simulink model "Table_airbus_v1"  (R2021b)
settings: Solver=VariableStepAuto  StartTime=0.0  StopTime=20  MaxStep=0.01  RelTol=0.01
undefined symbols (not defined in the file): X, Y, Z
libraries: sm_lib x907, fl_lib x69, nesl_utility x53, sdl_lib x10, ee_lib x7, slpidlib x6, simulink x5, simulink_extras x4
(part 2 of 18)

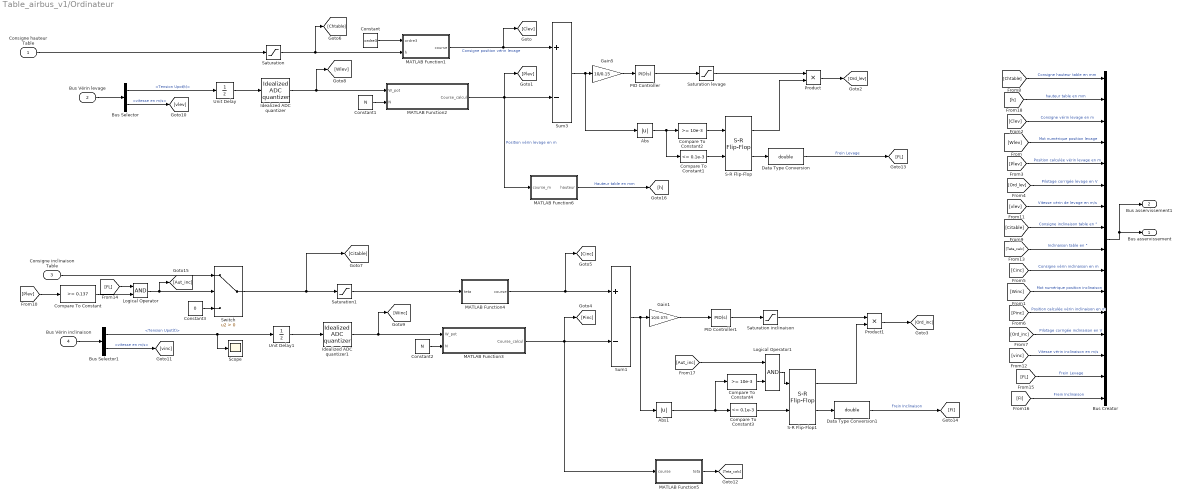
== system Table_airbus_v1/Ordinateur ==
  Consigne hauteur Table : Inport
  Bus Vérin levage : Inport  Port=2
  Consigne inclinaison Table : Inport  Port=3
  Bus Vérin inclinaison : Inport  Port=4
  Abs : Abs
  Abs1 : Abs
  Bus Creator : BusCreator  Inputs=16
  Bus Selector : BusSelector  OutputSignals=Tension Upot(t),Bus vis écrou.vitesse en m/s
  Bus Selector1 : BusSelector  OutputSignals=Tension Upot(t),Bus vis écrou.vitesse en m/s
  Compare To Constant : simulink/Logic and Bit Operations/Compare To Constant  relop=>=  const=0.137  OutDataTypeStr=boolean
  Compare To Constant1 : simulink/Logic and Bit Operations/Compare To Constant  relop=<=  const=0.1e-3  OutDataTypeStr=boolean
  Compare To Constant2 : simulink/Logic and Bit Operations/Compare To Constant  relop=>=  const=10e-3  OutDataTypeStr=boolean
  Compare To Constant3 : simulink/Logic and Bit Operations/Compare To Constant  relop=<=  const=0.1e-3  OutDataTypeStr=boolean
  Compare To Constant4 : simulink/Logic and Bit Operations/Compare To Constant  relop=>=  const=10e-3  OutDataTypeStr=boolean
  Constant : Constant  Value=ordre3
  Constant1 : Constant  Value=N
  Constant2 : Constant  Value=N
  Constant3 : Constant  Value=0
  Data Type Conversion : DataTypeConversion  OutDataTypeStr=double
  Data Type Conversion1 : DataTypeConversion  OutDataTypeStr=double
  Gain1 : Gain  Gain=10/0.075
  Gain5 : Gain  Gain=10/0.15
  Idealized ADC quantizer : simulink_extras/Additional Discrete/Idealized ADC quantizer  NumberOfConverterBits=N  Vmin=-10  Vmax=10  OutputDataType=int16  OutputNegativeValues=on
  Idealized ADC quantizer1 : simulink_extras/Additional Discrete/Idealized ADC quantizer  NumberOfConverterBits=N  Vmin=-10  Vmax=10  OutputDataType=int16  OutputNegativeValues=on
  Logical Operator : Logic  AllPortsSameDT=off  OutDataTypeStr=boolean
  Logical Operator1 : Logic  AllPortsSameDT=off  OutDataTypeStr=boolean
  MATLAB Function1 : MATLAB Function  TreatAsAtomicUnit=on
  MATLAB Function2 : MATLAB Function  TreatAsAtomicUnit=on
  MATLAB Function3 : MATLAB Function  TreatAsAtomicUnit=on
  MATLAB Function4 : MATLAB Function  TreatAsAtomicUnit=on
  MATLAB Function5 : MATLAB Function  TreatAsAtomicUnit=on
  MATLAB Function6 : MATLAB Function  TreatAsAtomicUnit=on
  PID Controller : slpidlib/PID Controller  Controller=PID  Form=Parallel  TimeDomain=Continuous-time  UseExternalTs=off  SampleTime=-1  IntegratorMethod=Forward Euler  FilterMethod=Forward Euler  ControllerParametersSource=internal  P=kp_lev  I=ki_lev  D=kd_lev  UseFilter=on  N=10  TunerSelectOption=Transfer Function Based (PID Tuner App)  InitialConditionSource=internal  InitialConditionForIntegrator=0  InitialConditionForFilter=0  DifferentiatorICPrevScaledInput=0  ExternalReset=none  TrackingMode=off  Kt=1  LimitOutput=off  SatLimitsSource=internal  UpperSaturationLimit=inf  LowerSaturationLimit=-inf  LinearizeAsGain=on  AntiWindupMode=none  Kb=1  POutMin=[]  POutMax=[]  IOutMin=[]  IOutMax=[]  DOutMin=[]  DOutMax=[]  NOutMin=[]  NOutMax=[]  SumOutMin=[]  SumOutMax=[]  SaturationOutMin=[]  SaturationOutMax=[]  PParamMin=[]  PParamMax=[]  IParamMin=[]  IParamMax=[]  DParamMin=[]  DParamMax=[]  NParamMin=[]  NParamMax=[]  KbParamMin=[]  KbParamMax=[]  KtParamMin=[]  KtParamMax=[]  KbOutMin=[]  KbOutMax=[]  KtOutMin=[]  KtOutMax=[]  IntegratorOutMin=[]  IntegratorOutMax=[]  FilterOutMin=[]  FilterOutMax=[]  SumI1OutMin=[]  SumI1OutMax=[]  SumI2OutMin=[]  SumI2OutMax=[]  SumI3OutMin=[]  SumI3OutMax=[]  SumI4OutMin=[]  SumI4OutMax=[]  SumDOutMin=[]  SumDOutMax=[]  DifferentiatorOutMin=[]  DifferentiatorOutMax=[]  FilterDiffOutCoefMin=[]  FilterDiffOutCoefMax=[]  ReciprocalOutMin=[]  ReciprocalOutMax=[]  SumDenOutMin=[]  SumDenOutMax=[]  SumNumOutMin=[]  SumNumOutMax=[]  DivideOutMin=[]  DivideOutMax=[]  UdiffTsProdOutMin=[]  UdiffTsProdOutMax=[]  NTsProdOutMin=[]  NTsProdOutMax=[]  UintegralTsProdOutMin=[]  UintegralTsProdOutMax=[]  UngainTsProdOutMin=[]  UngainTsProdOutMax=[]  IntegratorContinuousStateAttributes=''  IntegratorStateMustResolveToSignalObject=off  IntegratorRTWStateStorageClass=Auto  FilterContinuousStateAttributes=''  FilterStateMustResolveToSignalObject=off  FilterRTWStateStorageClass=Auto  ParallelPVariant=InternalParameters  IdealPVariant=Disabled  IVariant=InternalParameters  DVariant=InternalParameters  IntegratorVariant=Continuous  SatVariant=Disabled  AWVariant=Passthrough  PCopyVariant=Disabled  TRVariant=Disabled  FdbkBlocksVariant=Forward  IdealPFdbkVariant=Disabled  SatFdbkVariant=Disabled  DerivativeFilterVariant=ContFilter  NVariant=InternalParameters  NCopyVariant=Disabled  FilterICVariant=InternalICsFilter  IntegratorICVariant=InternalICs  ExternalResetVariant=Disabled  TRSumVariant=Passthrough  SumFdbkVariant=Disabled  SumVariant=Sum_PID  TsampFilterVariant=InternalTs  TsampNgainVariant=Passthrough  TsampIntegralVariant=Passthrough  ExternalSaturationOutDataTypeStr=Inherit: Same as second input
  PID Controller1 : slpidlib/PID Controller  Controller=PID  Form=Parallel  TimeDomain=Continuous-time  UseExternalTs=off  SampleTime=1  IntegratorMethod=Forward Euler  FilterMethod=Forward Euler  ControllerParametersSource=internal  P=kp_inc  I=ki_inc  D=kd_inc  UseFilter=on  N=10  TunerSelectOption=Transfer Function Based (PID Tuner App)  InitialConditionSource=internal  InitialConditionForIntegrator=0  InitialConditionForFilter=0  DifferentiatorICPrevScaledInput=0  ExternalReset=none  TrackingMode=off  Kt=1  LimitOutput=off  SatLimitsSource=internal  UpperSaturationLimit=inf  LowerSaturationLimit=-inf  LinearizeAsGain=on  AntiWindupMode=none  Kb=1  POutMin=[]  POutMax=[]  IOutMin=[]  IOutMax=[]  DOutMin=[]  DOutMax=[]  NOutMin=[]  NOutMax=[]  SumOutMin=[]  SumOutMax=[]  SaturationOutMin=[]  SaturationOutMax=[]  PParamMin=[]  PParamMax=[]  IParamMin=[]  IParamMax=[]  DParamMin=[]  DParamMax=[]  NParamMin=[]  NParamMax=[]  KbParamMin=[]  KbParamMax=[]  KtParamMin=[]  KtParamMax=[]  KbOutMin=[]  KbOutMax=[]  KtOutMin=[]  KtOutMax=[]  IntegratorOutMin=[]  IntegratorOutMax=[]  FilterOutMin=[]  FilterOutMax=[]  SumI1OutMin=[]  SumI1OutMax=[]  SumI2OutMin=[]  SumI2OutMax=[]  SumI3OutMin=[]  SumI3OutMax=[]  SumI4OutMin=[]  SumI4OutMax=[]  SumDOutMin=[]  SumDOutMax=[]  DifferentiatorOutMin=[]  DifferentiatorOutMax=[]  FilterDiffOutCoefMin=[]  FilterDiffOutCoefMax=[]  ReciprocalOutMin=[]  ReciprocalOutMax=[]  SumDenOutMin=[]  SumDenOutMax=[]  SumNumOutMin=[]  SumNumOutMax=[]  DivideOutMin=[]  DivideOutMax=[]  UdiffTsProdOutMin=[]  UdiffTsProdOutMax=[]  NTsProdOutMin=[]  NTsProdOutMax=[]  UintegralTsProdOutMin=[]  UintegralTsProdOutMax=[]  UngainTsProdOutMin=[]  UngainTsProdOutMax=[]  IntegratorContinuousStateAttributes=''  IntegratorStateMustResolveToSignalObject=off  IntegratorRTWStateStorageClass=Auto  FilterContinuousStateAttributes=''  FilterStateMustResolveToSignalObject=off  FilterRTWStateStorageClass=Auto  ParallelPVariant=InternalParameters  IdealPVariant=Disabled  IVariant=InternalParameters  DVariant=InternalParameters  IntegratorVariant=Continuous  SatVariant=Disabled  AWVariant=Passthrough  PCopyVariant=Disabled  TRVariant=Disabled  FdbkBlocksVariant=Forward  IdealPFdbkVariant=Disabled  SatFdbkVariant=Disabled  DerivativeFilterVariant=ContFilter  NVariant=InternalParameters  NCopyVariant=Disabled  FilterICVariant=InternalICsFilter  IntegratorICVariant=InternalICs  ExternalResetVariant=Disabled  TRSumVariant=Passthrough  SumFdbkVariant=Disabled  SumVariant=Sum_PID  TsampFilterVariant=InternalTs  TsampNgainVariant=Passthrough  TsampIntegralVariant=Passthrough  ExternalSaturationOutDataTypeStr=Inherit: Same as second input
  Product : Product
  Product1 : Product
  S-R Flip-Flop : simulink_extras/Flip Flops/S-R Flip-Flop  initial_condition=0
  S-R Flip-Flop1 : simulink_extras/Flip Flops/S-R Flip-Flop  initial_condition=0
  Saturation : Saturate  UpperLimit=pos_lev_max  LowerLimit=pos_lev_min
  Saturation inclinaison : Saturate  UpperLimit=10  LowerLimit=-10
  Saturation levage : Saturate  UpperLimit=10  LowerLimit=-10
  Saturation1 : Saturate  UpperLimit=20  LowerLimit=-20
  Scope : Scope
  Sum1 : Sum  Inputs=+-
  Sum3 : Sum  Inputs=+-
  Switch : Switch  Criteria=u2 > Threshold
  Unit Delay : UnitDelay  SampleTime=-1  HasFrameUpgradeWarning=on
  Unit Delay1 : UnitDelay  SampleTime=-1  HasFrameUpgradeWarning=on
  Bus asservissement : Outport  VectorParamsAs1DForOutWhenUnconnected=off
  Bus asservissement1 : Outport  Port=2  VectorParamsAs1DForOutWhenUnconnected=off
  wires:
  Saturation levage/1 -> Product/1
  Sum3/1 -> Abs/1, Gain5/1
  Consigne hauteur Table/1 -> Saturation/1
  MATLAB Function2/1(Course_calcul) -> MATLAB Function6/1(course_m), Sum3/2, [Plev]  "Position vérin levage en m"
  PID Controller/1 -> Saturation levage/1
  MATLAB Function3/1(Course_calcul) -> MATLAB Function5/1(course), [Pinc], Sum1/2
  MATLAB Function4/1(course) -> Sum1/1, [Cinc]
  Switch/1 -> [Citable], Saturation1/1
  Sum1/1 -> Abs1/1, Gain1/1
  MATLAB Function1/1(course) -> Sum3/1, [Clev]  "Consigne position vérin levage"
  Constant/1 -> MATLAB Function1/1(ordre3)
  Saturation/1 -> [Chtable], MATLAB Function1/2(h)
  [Clev] -> Bus Creator/3  "Consigne vérin levage en m"
  [Plev] -> Bus Creator/5  "Position calculée vérin levage en m"
  Bus Creator/1 -> Bus asservissement1/1, Bus asservissement/1
  [Ord_lev] -> Bus Creator/6  "Pilotage corrigée levage en V"
  [Ord_inc] -> Bus Creator/13  "Pilotage corrigée inclinaison en V"
  [Pinc] -> Bus Creator/12  "Position calculée vérin inclinaison en m"
  [Cinc] -> Bus Creator/10  "Consigne vérin inclinaison en m"
  [Chtable] -> Bus Creator/1  "Consigne hauteur table en mm"
  [Citable] -> Bus Creator/8  "Consigne inclinaison table en °"
  Bus Vérin inclinaison/1 -> Bus Selector1/1
  Constant1/1 -> MATLAB Function2/2(N)
  Gain5/1 -> PID Controller/1
  Constant2/1 -> MATLAB Function3/2(N)
  PID Controller1/1 -> Saturation inclinaison/1
  Gain1/1 -> PID Controller1/1
  Bus Selector1/1 -> Unit Delay1/1, Scope/1  "<Tension Upot(t)>"
  Bus Selector/1 -> Unit Delay/1  "<Tension Upot(t)>"
  Idealized ADC quantizer/1 -> [Wlev], MATLAB Function2/1(W_pot)
  [Wlev] -> Bus Creator/4  "Mot numérique position levage"
  Idealized ADC quantizer1/1 -> [Winc], MATLAB Function3/1(W_pot)
  Saturation1/1 -> MATLAB Function4/1(teta)
  [Winc] -> Bus Creator/11  "Mot numérique position inclinaison"
  [Plev] -> Compare To Constant/1
  Logical Operator/1 -> [Aut_inc], Switch/2
  Constant3/1 -> Switch/3
  Consigne inclinaison Table/1 -> Switch/1
  Unit Delay1/1 -> Idealized ADC quantizer1/1
  Bus Selector/2 -> [vlev]  "<vitesse en m/s>"
  [vlev] -> Bus Creator/7  "Vitesse vérin de levage en m/s"
  Unit Delay/1 -> Idealized ADC quantizer/1
  Bus Selector1/2 -> [vinc]  "<vitesse en m/s>"
  [vinc] -> Bus Creator/14  "Vitesse vérin inclinaison en m/s"
  MATLAB Function5/1(teta) -> [Teta_calc]
  [Teta_calc] -> Bus Creator/9  "Inclinaison table en °"
  Saturation inclinaison/1 -> Product1/1
  Data Type Conversion/1 -> [FL]  "Frein Levage"
  Compare To Constant2/1 -> S-R Flip-Flop/1
  Abs/1 -> Compare To Constant2/1, Compare To Constant1/1
  Bus Vérin levage/1 -> Bus Selector/1
  S-R Flip-Flop/2 -> Data Type Conversion/1
  Compare To Constant1/1 -> S-R Flip-Flop/2
  Product/1 -> [Ord_lev]
  S-R Flip-Flop/1 -> Product/2
  Compare To Constant/1 -> Logical Operator/2
  [FL] -> Logical Operator/1
  S-R Flip-Flop1/1 -> Product1/2
  S-R Flip-Flop1/2 -> Data Type Conversion1/1
  Data Type Conversion1/1 -> [FI]  "Frein Inclinaison"
  Product1/1 -> [Ord_inc]
  [FL] -> Bus Creator/15  "Frein Levage"
  [FI] -> Bus Creator/16  "Frein Inclinaison"
  [Aut_inc] -> Logical Operator1/1
  Abs1/1 -> Compare To Constant4/1, Compare To Constant3/1
  Compare To Constant3/1 -> S-R Flip-Flop1/2
  Logical Operator1/1 -> S-R Flip-Flop1/1
  Compare To Constant4/1 -> Logical Operator1/2
  MATLAB Function6/1(hauteur) -> [h]  "Hauteur table en mm"
  [h] -> Bus Creator/2  "hauteur table en mm"

== system Table_airbus_v1/Vérin électrique Inclinaison ==
  Pilotage Frein : Inport
  Bus Creator : BusCreator  Inputs=5
  Capteur : Subsystem
  Capteur mecanique Z1 : Subsystem
  Capteur mecanique Z2 : Subsystem
  Capteur mecanique Z3 : Subsystem
  Capteur mecanique Z4 : Subsystem
  Frein inclinaison : Subsystem
  Leadscrew : sdl_lib/Gears/Rotational- Translational/Leadscrew  Lead=pas_vis mm  helix_type=1  friction_model=2  friction_parameterization=1  lambda=Landa deg  alpha=Alpha deg  fr_coeff=fv  eff_sn=0.75  eff_ns=0.45  temperature_TLU=[280, 300, 320] K  efficiency_sn_TLU=[.75, .65, .6]  efficiency_ns_TLU=[.5, .45, .4]  pwr_thr=0.001 W  mu_visc=0 N*m/(rad/s)  thermal_mass=50 J/K  temperature_specify=off  temperature_priority=High  temperature=300 K  temperature_nominal_specify=off  temperature_nominal_unit=K  temperature_nominal_value=1
      settings: SourceProductBaseCode=LD  InternalSimscapePortConfiguration="{\"Bottom\":[],\"Left\":[{\"id\":\"S\",\"label\":\"S\",\"type\":\"foundation.mechanical.rotational.rotational\"}],\"Right\":[{\"id\":\"N\",\"label\":\"N\",\"type\":\"foundation.mechanical.translational.translational\"}],\"Top\":[]}"
  Mechanical Rotational Reference : fl_lib/Mechanical/Rotational Elements/Mechanical Rotational Reference
  Moteur : ee_lib/Electromechanical/Brushed Motors/DC Motor  field_option=ee.enum.field_option.pm  Rf=100 Ohm  Lf=1 H  Laf=0.15 H  If0=0 A  parameterization=1  Ra=R Ohm  La=L uH  emf_or_torque=2  Kv=0.0637 V/rpm  Ki=kt N*m/A  T_stall=3e-3*4000/(2*pi*6.25) N*m  w_max=3250 rpm  w_rated=2375 rpm  P_rated=19 W  V_rated=24 V  lam_param=2  i_noload=I0 A  V_i_noload=U0 V  J=Jm kg*m^2  lam=1e-08 N*m/(rad/s)  speed0=0 rpm  enable_fault_armature=simscape.enum.onoff.off  rev_faulted=1 / 3  G_faulted_armature=1e-5 S  fault_trigger_armature=ee.enum.faults.faultTrigger.temporal  t_fault_armature=1 s  max_permissible_current_armature=inf A  t_fail_on_current_armature=1 s  enable_fault_field=simscape.enum.onoff.off  G_faulted_field=1e-5 S  fault_trigger_field=ee.enum.faults.faultTrigger.temporal  t_fault_field=1 s  max_permissible_current_field=inf A  t_fail_on_current_field=1 s  fault_action=simscape.enum.assert.action.none  alpha=3.93e-3 1/K  Tmeas=25 degC  thermal_mass=100 J/K  initial_temperature=25 degC
  Scope : Scope
  réducteur train simple : sdl_lib/Gears/Simple Gear  ratio=ratio_red  rotation_direction=3-2*(1)  friction_model=sdl.enum.gear_efficiencies_load.constant  T_noload=0.1 N*m  T_nom=5 N*m  efficiency_nom=0.8  efficiency=rend_red/100  temperature_TLU=[280, 300, 320] K  load_TLU=[1, 5, 10] N*m  efficiency_TLU=[.95, .9, .85]  efficiency_TLU2=[.85, .8, .75; .95, .9, .85; .85, .8, .7]  w_thr=0.01 rad/s  pwr_thr=0.001 W  backlash_model=sdl.enum.backlashModel.Off  backlash_distance=1e-3 mm  x0=0 mm  r_base=0.1 m  hardstop_model=simscape.enum.hardstop.smooth  transition=1e-4 mm  backlash_stiffness=1e7 N/m  backlash_damping=1e6 N*s/m  e=0  v_tol=0.001 m/s  mu_visc=[0, 0] N*m/(rad/s)  enable_faults=simscape.enum.onoff.off  efficiency_fault=0.05  external_fault=simscape.enum.onoff.off  temporal_fault=simscape.enum.onoff.off  fault_time=5 s  fault_angles=pi / 12 rad  report_fault=(1)-1  thermal_mass=50 J/K  temperature_specify=off  temperature_priority=High  temperature=300 K  temperature_nominal_specify=off  temperature_nominal_unit=K  temperature_nominal_value=1  x_backlash_specify=off  x_backlash_priority=None  x_backlash=0 mm  x_backlash_nominal_specify=off  x_backlash_nominal_unit=mm  x_backlash_nominal_value=1  f_hardstop_specify=off  f_hardstop_priority=None  f_hardstop=0 N  f_hardstop_nominal_specify=off  f_hardstop_nominal_unit=N  f_hardstop_nominal_value=1  v_backlash_specify=off  v_backlash_priority=None  v_backlash=0 m/s  v_backlash_nominal_specify=off  v_backlash_nominal_unit=m/s  v_backlash_nominal_value=1
  réducteur train épicycloïdal : sdl_lib/Gears/Simple Gear  ratio=ratio_epi  rotation_direction=3-2*(1)  friction_model=sdl.enum.gear_efficiencies_load.constant  T_noload=0.1 N*m  T_nom=5 N*m  efficiency_nom=0.8  efficiency=rend_epi/100  temperature_TLU=[280, 300, 320] K  load_TLU=[1, 5, 10] N*m  efficiency_TLU=[.95, .9, .85]  efficiency_TLU2=[.85, .8, .75; .95, .9, .85; .85, .8, .7]  w_thr=0.01 rad/s  pwr_thr=0.001 W  backlash_model=sdl.enum.backlashModel.Off  backlash_distance=1e-3 mm  x0=0 mm  r_base=0.1 m  hardstop_model=simscape.enum.hardstop.smooth  transition=1e-4 mm  backlash_stiffness=1e7 N/m  backlash_damping=1e6 N*s/m  e=0  v_tol=0.001 m/s  mu_visc=[0, 0] N*m/(rad/s)  enable_faults=simscape.enum.onoff.off  efficiency_fault=0.05  external_fault=simscape.enum.onoff.off  temporal_fault=simscape.enum.onoff.off  fault_time=5 s  fault_angles=pi / 12 rad  report_fault=(1)-1  thermal_mass=50 J/K  temperature_specify=off  temperature_priority=High  temperature=300 K  temperature_nominal_specify=off  temperature_nominal_unit=K  temperature_nominal_value=1  x_backlash_specify=off  x_backlash_priority=None  x_backlash=0 mm  x_backlash_nominal_specify=off  x_backlash_nominal_unit=mm  x_backlash_nominal_value=1  f_hardstop_specify=off  f_hardstop_priority=None  f_hardstop=0 N  f_hardstop_nominal_specify=off  f_hardstop_nominal_unit=N  f_hardstop_nominal_value=1  v_backlash_specify=off  v_backlash_priority=None  v_backlash=0 m/s  v_backlash_nominal_specify=off  v_backlash_nominal_unit=m/s  v_backlash_nominal_value=1
  M+ : PMIOPort  Side=Left
  Tige : PMIOPort  Port=2  Side=Right
  M- : PMIOPort  Port=3  Side=Left
  Bus vérin Inclinaison : Outport  VectorParamsAs1DForOutWhenUnconnected=off
  wires:
  Pilotage Frein/1 -> Frein inclinaison/1(freinage), Scope/1
  [Bpot] -> Bus Creator/5  "Tension Upot(t)"
  Capteur/1(Upot) -> [Bpot]
  [Bve] -> Bus Creator/4  "Bus vis écrou"
  [Bts] -> Bus Creator/3  "Bus train simple"
  [Bte] -> Bus Creator/2  "Bus train epicycloïdal"
  Bus Creator/1 -> Bus vérin Inclinaison/1
  [Bmm] -> Bus Creator/1  "Bus meca moteur"
  Capteur mecanique Z2/1(Bus) -> [Bte]
  Capteur mecanique Z1/1(Bus) -> [Bmm]
  Capteur mecanique Z3/1(Bus) -> [Bts]
  Capteur mecanique Z4/1(Bus) -> [Bve]
  connections:
  Capteur/LConn1 -- Capteur mecanique Z4/RConn2
  Mechanical Rotational Reference/LConn1 -- Moteur/RConn2
  M-/RConn1 -- Moteur/RConn1
  M+/RConn1 -- Moteur/LConn1
  Capteur mecanique Z1/LConn1 -- Moteur/LConn2
  Capteur mecanique Z4/LConn1 -- Leadscrew/RConn1
  Leadscrew/LConn1 -- Capteur mecanique Z3/RConn1
  Capteur mecanique Z3/LConn1 -- réducteur train simple/RConn1
  réducteur train épicycloïdal/RConn1 -- Capteur mecanique Z2/LConn1
  Capteur mecanique Z1/RConn1 -- réducteur train épicycloïdal/LConn1
  Capteur mecanique Z4/RConn1 -- Tige/RConn1
  Capteur mecanique Z2/RConn1 -- réducteur train simple/LConn1 -- Frein inclinaison/RConn1

== system Table_airbus_v1/Vérin électrique Levage ==
  Pilotage Frein : Inport
  Bus Creator : BusCreator  Inputs=5
  Capteur : Subsystem
  Capteur mecanique Z1 : Subsystem
  Capteur mecanique Z2 : Subsystem
  Capteur mecanique Z3 : Subsystem
  Capteur mecanique Z4 : Subsystem
  Frein levage : Subsystem
  Leadscrew : sdl_lib/Gears/Rotational- Translational/Leadscrew  Lead=pas_vis mm  helix_type=1  friction_model=2  friction_parameterization=1  lambda=Landa deg  alpha=Alpha deg  fr_coeff=fv  eff_sn=0.75  eff_ns=0.45  temperature_TLU=[280, 300, 320] K  efficiency_sn_TLU=[.75, .65, .6]  efficiency_ns_TLU=[.5, .45, .4]  pwr_thr=0.001 W  mu_visc=0 N*m/(rad/s)  thermal_mass=50 J/K  temperature_specify=off  temperature_priority=High  temperature=300 K  temperature_nominal_specify=off  temperature_nominal_unit=K  temperature_nominal_value=1
      settings: SourceProductBaseCode=LD  InternalSimscapePortConfiguration="{\"Bottom\":[],\"Left\":[{\"id\":\"S\",\"label\":\"S\",\"type\":\"foundation.mechanical.rotational.rotational\"}],\"Right\":[{\"id\":\"N\",\"label\":\"N\",\"type\":\"foundation.mechanical.translational.translational\"}],\"Top\":[]}"
  Mechanical Rotational Reference : fl_lib/Mechanical/Rotational Elements/Mechanical Rotational Reference
  Moteur : ee_lib/Electromechanical/Brushed Motors/DC Motor  field_option=ee.enum.field_option.pm  Rf=100 Ohm  Lf=1 H  Laf=0.15 H  If0=0 A  parameterization=1  Ra=R Ohm  La=L uH  emf_or_torque=2  Kv=0.0637 V/rpm  Ki=kt N*m/A  T_stall=3e-3*4000/(2*pi*6.25) N*m  w_max=3250 rpm  w_rated=2375 rpm  P_rated=19 W  V_rated=24 V  lam_param=2  i_noload=I0 A  V_i_noload=U0 V  J=Jm kg*m^2  lam=1e-08 N*m/(rad/s)  speed0=0 rpm  enable_fault_armature=simscape.enum.onoff.off  rev_faulted=1 / 3  G_faulted_armature=1e-5 S  fault_trigger_armature=ee.enum.faults.faultTrigger.temporal  t_fault_armature=1 s  max_permissible_current_armature=inf A  t_fail_on_current_armature=1 s  enable_fault_field=simscape.enum.onoff.off  G_faulted_field=1e-5 S  fault_trigger_field=ee.enum.faults.faultTrigger.temporal  t_fault_field=1 s  max_permissible_current_field=inf A  t_fail_on_current_field=1 s  fault_action=simscape.enum.assert.action.none  alpha=3.93e-3 1/K  Tmeas=25 degC  thermal_mass=100 J/K  initial_temperature=25 degC
  Scope : Scope
  réducteur train simple : sdl_lib/Gears/Simple Gear  ratio=ratio_red  rotation_direction=3-2*(1)  friction_model=sdl.enum.gear_efficiencies_load.constant  T_noload=0.1 N*m  T_nom=5 N*m  efficiency_nom=0.8  efficiency=rend_red/100  temperature_TLU=[280, 300, 320] K  load_TLU=[1, 5, 10] N*m  efficiency_TLU=[.95, .9, .85]  efficiency_TLU2=[.85, .8, .75; .95, .9, .85; .85, .8, .7]  w_thr=0.01 rad/s  pwr_thr=0.001 W  backlash_model=sdl.enum.backlashModel.Off  backlash_distance=1e-3 mm  x0=0 mm  r_base=0.1 m  hardstop_model=simscape.enum.hardstop.smooth  transition=1e-4 mm  backlash_stiffness=1e7 N/m  backlash_damping=1e6 N*s/m  e=0  v_tol=0.001 m/s  mu_visc=[0, 0] N*m/(rad/s)  enable_faults=simscape.enum.onoff.off  efficiency_fault=0.05  external_fault=simscape.enum.onoff.off  temporal_fault=simscape.enum.onoff.off  fault_time=5 s  fault_angles=pi / 12 rad  report_fault=(1)-1  thermal_mass=50 J/K  temperature_specify=off  temperature_priority=High  temperature=300 K  temperature_nominal_specify=off  temperature_nominal_unit=K  temperature_nominal_value=1  x_backlash_specify=off  x_backlash_priority=None  x_backlash=0 mm  x_backlash_nominal_specify=off  x_backlash_nominal_unit=mm  x_backlash_nominal_value=1  f_hardstop_specify=off  f_hardstop_priority=None  f_hardstop=0 N  f_hardstop_nominal_specify=off  f_hardstop_nominal_unit=N  f_hardstop_nominal_value=1  v_backlash_specify=off  v_backlash_priority=None  v_backlash=0 m/s  v_backlash_nominal_specify=off  v_backlash_nominal_unit=m/s  v_backlash_nominal_value=1
  réducteur train épicycloïdal : sdl_lib/Gears/Simple Gear  ratio=ratio_epi  rotation_direction=3-2*(1)  friction_model=sdl.enum.gear_efficiencies_load.constant  T_noload=0.1 N*m  T_nom=5 N*m  efficiency_nom=0.8  efficiency=rend_epi/100  temperature_TLU=[280, 300, 320] K  load_TLU=[1, 5, 10] N*m  efficiency_TLU=[.95, .9, .85]  efficiency_TLU2=[.85, .8, .75; .95, .9, .85; .85, .8, .7]  w_thr=0.01 rad/s  pwr_thr=0.001 W  backlash_model=sdl.enum.backlashModel.Off  backlash_distance=1e-3 mm  x0=0 mm  r_base=0.1 m  hardstop_model=simscape.enum.hardstop.smooth  transition=1e-4 mm  backlash_stiffness=1e7 N/m  backlash_damping=1e6 N*s/m  e=0  v_tol=0.001 m/s  mu_visc=[0, 0] N*m/(rad/s)  enable_faults=simscape.enum.onoff.off  efficiency_fault=0.05  external_fault=simscape.enum.onoff.off  temporal_fault=simscape.enum.onoff.off  fault_time=5 s  fault_angles=pi / 12 rad  report_fault=(1)-1  thermal_mass=50 J/K  temperature_specify=off  temperature_priority=High  temperature=300 K  temperature_nominal_specify=off  temperature_nominal_unit=K  temperature_nominal_value=1  x_backlash_specify=off  x_backlash_priority=None  x_backlash=0 mm  x_backlash_nominal_specify=off  x_backlash_nominal_unit=mm  x_backlash_nominal_value=1  f_hardstop_specify=off  f_hardstop_priority=None  f_hardstop=0 N  f_hardstop_nominal_specify=off  f_hardstop_nominal_unit=N  f_hardstop_nominal_value=1  v_backlash_specify=off  v_backlash_priority=None  v_backlash=0 m/s  v_backlash_nominal_specify=off  v_backlash_nominal_unit=m/s  v_backlash_nominal_value=1
  M+ : PMIOPort  Side=Left
  Tige : PMIOPort  Port=2  Side=Right
  M- : PMIOPort  Port=3  Side=Left
  Bus vérin levage : Outport  VectorParamsAs1DForOutWhenUnconnected=off
  wires:
  Capteur mecanique Z4/1(Bus) -> [Bve]
  Capteur mecanique Z3/1(Bus) -> [Bts]
  Capteur mecanique Z1/1(Bus) -> [Bmm]
  Capteur mecanique Z2/1(Bus) -> [Bte]
  [Bmm] -> Bus Creator/1  "Bus meca moteur"
  Bus Creator/1 -> Bus vérin levage/1
  [Bte] -> Bus Creator/2  "Bus train epicycloïdal"
  [Bts] -> Bus Creator/3  "Bus train simple"
  [Bve] -> Bus Creator/4  "Bus vis écrou"
  Capteur/1(Upot) -> [Bpot]
  [Bpot] -> Bus Creator/5  "Tension Upot(t)"
  Pilotage Frein/1 -> Scope/1, Frein levage/1(freinage)
  connections:
  Frein levage/RConn1 -- réducteur train simple/LConn1 -- Capteur mecanique Z2/RConn1
  Capteur mecanique Z4/RConn1 -- Tige/RConn1
  Capteur mecanique Z1/RConn1 -- réducteur train épicycloïdal/LConn1
  réducteur train épicycloïdal/RConn1 -- Capteur mecanique Z2/LConn1
  Capteur mecanique Z3/LConn1 -- réducteur train simple/RConn1
  Leadscrew/LConn1 -- Capteur mecanique Z3/RConn1
  Capteur mecanique Z4/LConn1 -- Leadscrew/RConn1
  Capteur mecanique Z1/LConn1 -- Moteur/LConn2
  M+/RConn1 -- Moteur/LConn1
  M-/RConn1 -- Moteur/RConn1
  Mechanical Rotational Reference/LConn1 -- Moteur/RConn2
  Capteur/LConn1 -- Capteur mecanique Z4/RConn2

== system Table_airbus_v1/Alimentation/Capteur électrique alim ==
  Bus Creator : BusCreator  Inputs=3
  Current Sensor1 : fl_lib/Electrical/Electrical Sensors/Current Sensor
  PS-Simulink1 : nesl_utility/PS-Simulink Converter  PhysicalDomain=network_engine_domain  SubClassName=ps_output  LeftPortType=input  RightPortType=output  PseudoPeriodic=off  Frequencies=[]  Unit=V  AffineConversion=off
      settings: SourceProductBaseCode=PW,SS
  PS-Simulink4 : nesl_utility/PS-Simulink Converter  PhysicalDomain=network_engine_domain  SubClassName=ps_output  LeftPortType=input  RightPortType=output  PseudoPeriodic=off  Frequencies=[]  Unit=A  AffineConversion=off
      settings: SourceProductBaseCode=PW,SS
  Product : Product
  Voltage Sensor : fl_lib/Electrical/Electrical Sensors/Voltage Sensor
  S+ : PMIOPort  Side=Right
  E+ : PMIOPort  Port=2  Side=Left
  E- : PMIOPort  Port=3  Side=Left
  S- : PMIOPort  Port=4  Side=Right
  Bus : Outport  VectorParamsAs1DForOutWhenUnconnected=off
  wires:
  PS-Simulink1/1 -> Bus Creator/2, Product/2  "tension en V"
  PS-Simulink4/1 -> Bus Creator/1, Product/1  "Intensité A"
  Bus Creator/1 -> Bus/1
  Product/1 -> Bus Creator/3  "puissance en W"
  connections:
  E-/RConn1 -- Voltage Sensor/RConn2 -- S-/RConn1
  Voltage Sensor/LConn1 -- Current Sensor1/RConn2 -- S+/RConn1
  E+/RConn1 -- Current Sensor1/LConn1
  PS-Simulink4/LConn1 -- Current Sensor1/RConn1
  PS-Simulink1/LConn1 -- Voltage Sensor/RConn1

== system Table_airbus_v1/Hacheur 4 Quadrants Unipolaire moyen Inc/Hacheur 4 Q ==
  Pilotage Hacheur : Inport
  Capteur électrique hacheur : Subsystem
  Constant : Constant  Value=Vd
  Constant1 : Constant  Value=Rd
  Constant2 : Constant  Value=Rds
  Controlled Current Source : fl_lib/Electrical/Electrical Sources/Controlled Current Source
  Controlled Voltage Source : fl_lib/Electrical/Electrical Sources/Controlled Voltage Source
  Controlled Voltage Source1 : fl_lib/Electrical/Electrical Sources/Controlled Voltage Source
  Current Sensor : fl_lib/Electrical/Electrical Sensors/Current Sensor
  Electrical Reference Continu : fl_lib/Electrical/Electrical Elements/Electrical Reference
  MATLAB Function : MATLAB Function  TreatAsAtomicUnit=on
  PS-Simulink Converter : nesl_utility/PS-Simulink Converter  PhysicalDomain=network_engine_domain  SubClassName=ps_output  LeftPortType=input  RightPortType=output  PseudoPeriodic=off  Frequencies=[]  Unit=V  AffineConversion=off
      settings: SourceProductBaseCode=PW,SS
  PS-Simulink Converter1 : nesl_utility/PS-Simulink Converter  PhysicalDomain=network_engine_domain  SubClassName=ps_output  LeftPortType=input  RightPortType=output  PseudoPeriodic=off  Frequencies=[]  Unit=A  AffineConversion=off
      settings: SourceProductBaseCode=PW,SS
  Product : Product
  Product1 : Product
  Scope : Scope  NumInputPorts=3
  Simulink-PS Converter1 : nesl_utility/Simulink-PS Converter  PhysicalDomain=network_engine_domain  SubClassName=ps_input  LeftPortType=input  RightPortType=output  PseudoPeriodic=off  Frequencies=[]  NoiseDistribution=none  NoiseParameters=[]  Unit=Ohm  AffineConversion=off  FilteringAndDerivatives=zero  SimscapeFilterOrder=1  InputFilterTimeConstant=0.001  UdotUserProvided=1
      settings: SourceProductBaseCode=PW,SS
  Simulink-PS Converter2 : nesl_utility/Simulink-PS Converter  PhysicalDomain=network_engine_domain  SubClassName=ps_input  LeftPortType=input  RightPortType=output  PseudoPeriodic=off  Frequencies=[]  NoiseDistribution=none  NoiseParameters=[]  Unit=V  AffineConversion=off  FilteringAndDerivatives=zero  SimscapeFilterOrder=1  InputFilterTimeConstant=0.001  UdotUserProvided=1
      settings: SourceProductBaseCode=PW,SS
  Simulink-PS Converter3 : nesl_utility/Simulink-PS Converter  PhysicalDomain=network_engine_domain  SubClassName=ps_input  LeftPortType=input  RightPortType=output  PseudoPeriodic=off  Frequencies=[]  NoiseDistribution=none  NoiseParameters=[]  Unit=V  AffineConversion=off  FilteringAndDerivatives=zero  SimscapeFilterOrder=1  InputFilterTimeConstant=0.001  UdotUserProvided=1
      settings: SourceProductBaseCode=PW,SS
  Simulink-PS Converter4 : nesl_utility/Simulink-PS Converter  PhysicalDomain=network_engine_domain  SubClassName=ps_input  LeftPortType=input  RightPortType=output  PseudoPeriodic=off  Frequencies=[]  NoiseDistribution=none  NoiseParameters=[]  Unit=A  AffineConversion=off  FilteringAndDerivatives=zero  SimscapeFilterOrder=1  InputFilterTimeConstant=0.001  UdotUserProvided=1
      settings: SourceProductBaseCode=PW,SS
  Variable Resistor : fl_lib/Electrical/Electrical Elements/Variable Resistor  Rmin=0 Ohm  i_specify=off  i_priority=None  i=0 A  i_nominal_specify=off  i_nominal_unit=A  i_nominal_value=1  v_specify=off  v_priority=None  v=0 V  v_nominal_specify=off  v_nominal_unit=V  v_nominal_value=1
  Voltage Sensor : fl_lib/Electrical/Electrical Sensors/Voltage Sensor
  E+ : PMIOPort  Side=Left
  M+ : PMIOPort  Port=2  Side=Right
  E- : PMIOPort  Port=3  Side=Left
  M- : PMIOPort  Port=4  Side=Right
  Bus_mesure_hacheur : Outport  VectorParamsAs1DForOutWhenUnconnected=off
  wires:
  Pilotage Hacheur/1 -> MATLAB Function/4(alpha), Product1/2, Product/1, Scope/1
  PS-Simulink Converter1/1 -> Product1/1
  Product1/1 -> Simulink-PS Converter4/1
  PS-Simulink Converter/1 -> Product/2
  Product/1 -> Simulink-PS Converter3/1
  Constant2/1 -> MATLAB Function/1(Rds)
  Constant1/1 -> MATLAB Function/2(Rd)
  Constant/1 -> MATLAB Function/3(Vd)
  MATLAB Function/2(Vhach) -> Simulink-PS Converter2/1, Scope/3
  MATLAB Function/1(Rhach) -> Simulink-PS Converter1/1, Scope/2
  Capteur électrique hacheur/1(Bus) -> Bus_mesure_hacheur/1  "Bus_mesure_hacheur"
  connections:
  Variable Resistor/RConn1 -- Capteur électrique hacheur/LConn1
  Controlled Voltage Source1/RConn2 -- Current Sensor/RConn2
  PS-Simulink Converter1/LConn1 -- Current Sensor/RConn1
  Simulink-PS Converter4/RConn1 -- Controlled Current Source/RConn1
  PS-Simulink Converter/LConn1 -- Voltage Sensor/RConn1
  Simulink-PS Converter3/RConn1 -- Controlled Voltage Source/RConn1
  Simulink-PS Converter2/RConn1 -- Controlled Voltage Source1/RConn1
  Simulink-PS Converter1/RConn1 -- Variable Resistor/LConn1
  Controlled Voltage Source1/LConn1 -- Variable Resistor/LConn2
  M+/RConn1 -- Capteur électrique hacheur/RConn1
  Voltage Sensor/LConn1 -- E+/RConn1 -- Controlled Current Source/RConn2
  Current Sensor/LConn1 -- Controlled Voltage Source/LConn1
  Voltage Sensor/RConn2 -- E-/RConn1 -- Controlled Current Source/LConn1
  Controlled Voltage Source/RConn2 -- Electrical Reference Continu/LConn1 -- M-/RConn1 -- Capteur électrique hacheur/LConn2

== system Table_airbus_v1/Hacheur 4 Quadrants Unipolaire moyen lev/Hacheur 4 Q ==
  Pilotage Hacheur : Inport
  Capteur électrique hacheur : Subsystem
  Constant : Constant  Value=Vd
  Constant1 : Constant  Value=Rd
  Constant2 : Constant  Value=Rds
  Controlled Current Source : fl_lib/Electrical/Electrical Sources/Controlled Current Source
  Controlled Voltage Source : fl_lib/Electrical/Electrical Sources/Controlled Voltage Source
  Controlled Voltage Source1 : fl_lib/Electrical/Electrical Sources/Controlled Voltage Source
  Current Sensor : fl_lib/Electrical/Electrical Sensors/Current Sensor
  Electrical Reference Continu : fl_lib/Electrical/Electrical Elements/Electrical Reference
  MATLAB Function : MATLAB Function  TreatAsAtomicUnit=on
  PS-Simulink Converter : nesl_utility/PS-Simulink Converter  PhysicalDomain=network_engine_domain  SubClassName=ps_output  LeftPortType=input  RightPortType=output  PseudoPeriodic=off  Frequencies=[]  Unit=V  AffineConversion=off
      settings: SourceProductBaseCode=PW,SS
  PS-Simulink Converter1 : nesl_utility/PS-Simulink Converter  PhysicalDomain=network_engine_domain  SubClassName=ps_output  LeftPortType=input  RightPortType=output  PseudoPeriodic=off  Frequencies=[]  Unit=A  AffineConversion=off
      settings: SourceProductBaseCode=PW,SS
  Product : Product
  Product1 : Product
  Scope : Scope  NumInputPorts=3
  Simulink-PS Converter1 : nesl_utility/Simulink-PS Converter  PhysicalDomain=network_engine_domain  SubClassName=ps_input  LeftPortType=input  RightPortType=output  PseudoPeriodic=off  Frequencies=[]  NoiseDistribution=none  NoiseParameters=[]  Unit=Ohm  AffineConversion=off  FilteringAndDerivatives=zero  SimscapeFilterOrder=1  InputFilterTimeConstant=0.001  UdotUserProvided=1
      settings: SourceProductBaseCode=PW,SS
  Simulink-PS Converter2 : nesl_utility/Simulink-PS Converter  PhysicalDomain=network_engine_domain  SubClassName=ps_input  LeftPortType=input  RightPortType=output  PseudoPeriodic=off  Frequencies=[]  NoiseDistribution=none  NoiseParameters=[]  Unit=V  AffineConversion=off  FilteringAndDerivatives=zero  SimscapeFilterOrder=1  InputFilterTimeConstant=0.001  UdotUserProvided=1
      settings: SourceProductBaseCode=PW,SS
  Simulink-PS Converter3 : nesl_utility/Simulink-PS Converter  PhysicalDomain=network_engine_domain  SubClassName=ps_input  LeftPortType=input  RightPortType=output  PseudoPeriodic=off  Frequencies=[]  NoiseDistribution=none  NoiseParameters=[]  Unit=V  AffineConversion=off  FilteringAndDerivatives=zero  SimscapeFilterOrder=1  InputFilterTimeConstant=0.001  UdotUserProvided=1
      settings: SourceProductBaseCode=PW,SS
  Simulink-PS Converter4 : nesl_utility/Simulink-PS Converter  PhysicalDomain=network_engine_domain  SubClassName=ps_input  LeftPortType=input  RightPortType=output  PseudoPeriodic=off  Frequencies=[]  NoiseDistribution=none  NoiseParameters=[]  Unit=A  AffineConversion=off  FilteringAndDerivatives=zero  SimscapeFilterOrder=1  InputFilterTimeConstant=0.001  UdotUserProvided=1
      settings: SourceProductBaseCode=PW,SS
  Variable Resistor : fl_lib/Electrical/Electrical Elements/Variable Resistor  Rmin=0 Ohm  i_specify=off  i_priority=None  i=0 A  i_nominal_specify=off  i_nominal_unit=A  i_nominal_value=1  v_specify=off  v_priority=None  v=0 V  v_nominal_specify=off  v_nominal_unit=V  v_nominal_value=1
  Voltage Sensor : fl_lib/Electrical/Electrical Sensors/Voltage Sensor
  E+ : PMIOPort  Side=Left
  M+ : PMIOPort  Port=2  Side=Right
  E- : PMIOPort  Port=3  Side=Left
  M- : PMIOPort  Port=4  Side=Right
  Bus_mesure_hacheur : Outport  VectorParamsAs1DForOutWhenUnconnected=off
  wires:
  Capteur électrique hacheur/1(Bus) -> Bus_mesure_hacheur/1  "Bus_mesure_hacheur"
  MATLAB Function/1(Rhach) -> Scope/2, Simulink-PS Converter1/1
  MATLAB Function/2(Vhach) -> Scope/3, Simulink-PS Converter2/1
  Constant/1 -> MATLAB Function/3(Vd)
  Constant1/1 -> MATLAB Function/2(Rd)
  Constant2/1 -> MATLAB Function/1(Rds)
  Product/1 -> Simulink-PS Converter3/1
  PS-Simulink Converter/1 -> Product/2
  Product1/1 -> Simulink-PS Converter4/1
  PS-Simulink Converter1/1 -> Product1/1
  Pilotage Hacheur/1 -> Scope/1, Product/1, Product1/2, MATLAB Function/4(alpha)
  connections:
  Capteur électrique hacheur/LConn2 -- M-/RConn1 -- Electrical Reference Continu/LConn1 -- Controlled Voltage Source/RConn2
  Controlled Current Source/LConn1 -- E-/RConn1 -- Voltage Sensor/RConn2
  Current Sensor/LConn1 -- Controlled Voltage Source/LConn1
  Controlled Current Source/RConn2 -- E+/RConn1 -- Voltage Sensor/LConn1
  M+/RConn1 -- Capteur électrique hacheur/RConn1
  Controlled Voltage Source1/LConn1 -- Variable Resistor/LConn2
  Simulink-PS Converter1/RConn1 -- Variable Resistor/LConn1
  Simulink-PS Converter2/RConn1 -- Controlled Voltage Source1/RConn1
  Simulink-PS Converter3/RConn1 -- Controlled Voltage Source/RConn1
  PS-Simulink Converter/LConn1 -- Voltage Sensor/RConn1
  Simulink-PS Converter4/RConn1 -- Controlled Current Source/RConn1
  PS-Simulink Converter1/LConn1 -- Current Sensor/RConn1
  Controlled Voltage Source1/RConn2 -- Current Sensor/RConn2
  Variable Resistor/RConn1 -- Capteur électrique hacheur/LConn1

== system Table_airbus_v1/Modèle mécanique/Passerelle Simscape transaltion levage ==
  Ideal Force Sensor : fl_lib/Mechanical/Mechanical Sensors/Ideal Force Sensor
  Ideal Translational Velocity Source : fl_lib/Mechanical/Mechanical Sources/Ideal Translational Velocity Source
  Tige verin : PMIOPort  Side=Left
  Corps verin : PMIOPort  Port=2  Side=Left
  V : PMIOPort  Port=3  Side=Right
  Fm : PMIOPort  Port=4  Side=Right
  connections:
  Tige verin/RConn1 -- Ideal Force Sensor/LConn1
  Ideal Translational Velocity Source/LConn1 -- Ideal Force Sensor/RConn1
  Ideal Translational Velocity Source/RConn2 -- Corps verin/RConn1
  Fm/RConn1 -- Ideal Force Sensor/RConn2
  V/RConn1 -- Ideal Translational Velocity Source/RConn1

== system Table_airbus_v1/Modèle mécanique/Passerelle Simscape translation inclinaison ==
  Ideal Force Sensor : fl_lib/Mechanical/Mechanical Sensors/Ideal Force Sensor
  Ideal Translational Velocity Source : fl_lib/Mechanical/Mechanical Sources/Ideal Translational Velocity Source
  Tige verin : PMIOPort  Side=Left
  Corps verin : PMIOPort  Port=2  Side=Left
  Fm : PMIOPort  Port=3  Side=Right
  V : PMIOPort  Port=4  Side=Right
  connections:
  V/RConn1 -- Ideal Translational Velocity Source/RConn1
  Fm/RConn1 -- Ideal Force Sensor/RConn2
  Ideal Translational Velocity Source/RConn2 -- Corps verin/RConn1
  Ideal Translational Velocity Source/LConn1 -- Ideal Force Sensor/RConn1
  Tige verin/RConn1 -- Ideal Force Sensor/LConn1
